simulink model "pend2"  (R2017b)
settings: Solver=VariableStepAuto  StartTime=0.0  StopTime=1  RelTol=1e-3
libraries: simulink_extras x6, simulink x2
settings Model: Creator=Iman  LastModifiedBy=Iman

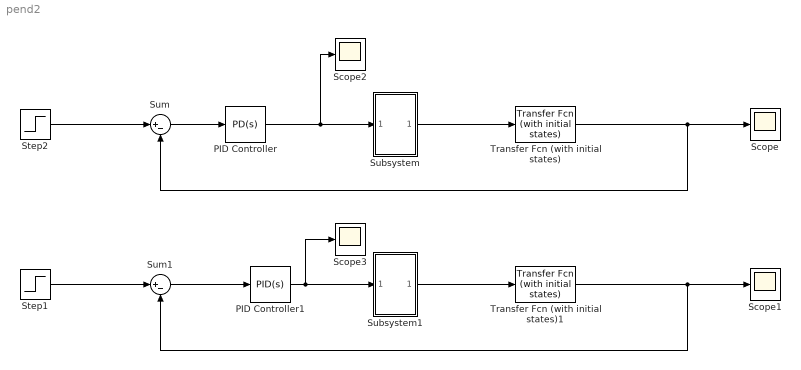
== system pend2 ==
  PID Controller : simulink/Continuous/PID Controller  Controller=PD  TimeDomain=Continuous-time  SampleTime=-1  IntegratorMethod=Forward Euler  FilterMethod=Forward Euler  Form=Parallel  UseFilter=on  ControllerParametersSource=internal  P=-1149.38229083247  I=-498.232243634702  D=-2.84895426178674  N=145.911718528072  InitialConditionSource=internal  InitialConditionForIntegrator=0  InitialConditionForFilter=0  ExternalReset=none  LimitOutput=off  UpperSaturationLimit=inf  LowerSaturationLimit=-inf  LinearizeAsGain=on  AntiWindupMode=none  Kb=1  TrackingMode=off  Kt=1  PParamMin=[]  PParamMax=[]  IParamMin=[]  IParamMax=[]  DParamMin=[]  DParamMax=[]  NParamMin=[]  NParamMax=[]  KbParamMin=[]  KbParamMax=[]  KtParamMin=[]  KtParamMax=[]  POutMin=[]  POutMax=[]  IOutMin=[]  IOutMax=[]  DOutMin=[]  DOutMax=[]  NOutMin=[]  NOutMax=[]  KbOutMin=[]  KbOutMax=[]  KtOutMin=[]  KtOutMax=[]  IntegratorOutMin=[]  IntegratorOutMax=[]  FilterOutMin=[]  FilterOutMax=[]  SumOutMin=[]  SumOutMax=[]  SumI1OutMin=[]  SumI1OutMax=[]  SumI2OutMin=[]  SumI2OutMax=[]  SumI3OutMin=[]  SumI3OutMax=[]  SumDOutMin=[]  SumDOutMax=[]  SaturationOutMin=[]  SaturationOutMax=[]  IntegratorContinuousStateAttributes=''  IntegratorStateMustResolveToSignalObject=off  IntegratorRTWStateStorageClass=Auto  FilterContinuousStateAttributes=''  FilterStateMustResolveToSignalObject=off  FilterRTWStateStorageClass=Auto  DifferentiatorICPrevScaledInput=0  DifferentiatorOutMin=[]  DifferentiatorOutMax=[]  InitialConditionSetting=State (most efficient)  FilterDiffOutCoefMin=[]  FilterDiffOutCoefMax=[]  SumDenOutMin=[]  SumDenOutMax=[]  SumNumOutMin=[]  SumNumOutMax=[]  ReciprocalOutMin=[]  ReciprocalOutMax=[]  DivideOutMin=[]  DivideOutMax=[]  TunerSelectOption=Transfer Function Based (PID Tuner App)
  PID Controller1 : simulink/Continuous/PID Controller  Controller=PID  TimeDomain=Continuous-time  SampleTime=-1  IntegratorMethod=Forward Euler  FilterMethod=Forward Euler  Form=Parallel  UseFilter=on  ControllerParametersSource=internal  P=50303643.3579245  I=36418344513.5141  D=15438.3063033628  N=14182098.2865599  InitialConditionSource=internal  InitialConditionForIntegrator=0  InitialConditionForFilter=0  ExternalReset=none  LimitOutput=off  UpperSaturationLimit=inf  LowerSaturationLimit=-inf  LinearizeAsGain=on  AntiWindupMode=none  Kb=1  TrackingMode=off  Kt=1  PParamMin=[]  PParamMax=[]  IParamMin=[]  IParamMax=[]  DParamMin=[]  DParamMax=[]  NParamMin=[]  NParamMax=[]  KbParamMin=[]  KbParamMax=[]  KtParamMin=[]  KtParamMax=[]  POutMin=[]  POutMax=[]  IOutMin=[]  IOutMax=[]  DOutMin=[]  DOutMax=[]  NOutMin=[]  NOutMax=[]  KbOutMin=[]  KbOutMax=[]  KtOutMin=[]  KtOutMax=[]  IntegratorOutMin=[]  IntegratorOutMax=[]  FilterOutMin=[]  FilterOutMax=[]  SumOutMin=[]  SumOutMax=[]  SumI1OutMin=[]  SumI1OutMax=[]  SumI2OutMin=[]  SumI2OutMax=[]  SumI3OutMin=[]  SumI3OutMax=[]  SumDOutMin=[]  SumDOutMax=[]  SaturationOutMin=[]  SaturationOutMax=[]  IntegratorContinuousStateAttributes=''  IntegratorStateMustResolveToSignalObject=off  IntegratorRTWStateStorageClass=Auto  FilterContinuousStateAttributes=''  FilterStateMustResolveToSignalObject=off  FilterRTWStateStorageClass=Auto  DifferentiatorICPrevScaledInput=0  DifferentiatorOutMin=[]  DifferentiatorOutMax=[]  InitialConditionSetting=State (most efficient)  FilterDiffOutCoefMin=[]  FilterDiffOutCoefMax=[]  SumDenOutMin=[]  SumDenOutMax=[]  SumNumOutMin=[]  SumNumOutMax=[]  ReciprocalOutMin=[]  ReciprocalOutMax=[]  DivideOutMin=[]  DivideOutMax=[]  TunerSelectOption=Transfer Function Based (PID Tuner App)
  Scope{,1..3} (4 alike) : Scope
  Step1 : Step  Time=0  SampleTime=0.1
  Step2 : Step  Time=0  After=0.01  SampleTime=0.1
  Subsystem : Subsystem
  Subsystem1 : Subsystem
  Sum : Sum  Inputs=|+-
  Sum1 : Sum  Inputs=|+-
  Transfer Fcn (with initial states) : simulink_extras/Additional Linear/Transfer Fcn (with initial states)  N=[-1374 -7.66e04]  D=[1 2549 -370.1 -1.28e05]  X0=0
  Transfer Fcn (with initial states)1 : simulink_extras/Additional Linear/Transfer Fcn (with initial states)  N=[104.5 -3064 -6898]  D=[1 2549 -370.1 -1.28e05 0]  X0=0
  wires:
  Transfer Fcn (with initial states)/1 -> Sum/2, Scope/1
  Step2/1 -> Sum/1
  Sum/1 -> PID Controller/1
  PID Controller/1 -> Scope2/1, Subsystem/1(In1)
  Subsystem/1(Out1) -> Transfer Fcn (with initial states)/1
  Transfer Fcn (with initial states)1/1 -> Sum1/2, Scope1/1
  PID Controller1/1 -> Scope3/1, Subsystem1/1(In1)
  Subsystem1/1(Out1) -> Transfer Fcn (with initial states)1/1
  Step1/1 -> Sum1/1
  Sum1/1 -> PID Controller1/1

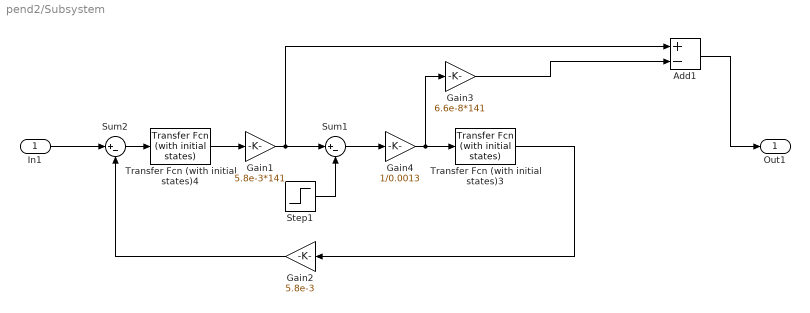
== system pend2/Subsystem ==
  In1 : Inport
  Add1 : Sum  Inputs=+-
  Gain1 : Gain  Gain=5.8e-3*141
  Gain2 : Gain  Gain=5.8e-3
  Gain3 : Gain  Gain=6.6e-8*141
  Gain4 : Gain  Gain=1/0.0013
  Step1 : Step  Time=0  SampleTime=0.1
  Sum1 : Sum  Inputs=|+-
  Sum2 : Sum  Inputs=|+-
  Transfer Fcn (with initial states)3 : simulink_extras/Additional Linear/Transfer Fcn (with initial states)  N=[1]  D=[1 0]  X0=0
  Transfer Fcn (with initial states)4 : simulink_extras/Additional Linear/Transfer Fcn (with initial states)  N=[1]  D=[7e-5 6]  X0=0
  Out1 : Outport
  wires:
  Transfer Fcn (with initial states)3/1 -> Gain2/1
  Step1/1 -> Sum1/2
  Sum1/1 -> Gain4/1
  Add1/1 -> Out1/1
  Gain1/1 -> Sum1/1, Add1/1
  Gain2/1 -> Sum2/2
  Transfer Fcn (with initial states)4/1 -> Gain1/1
  Gain3/1 -> Add1/2
  Gain4/1 -> Gain3/1, Transfer Fcn (with initial states)3/1
  Sum2/1 -> Transfer Fcn (with initial states)4/1
  In1/1 -> Sum2/1

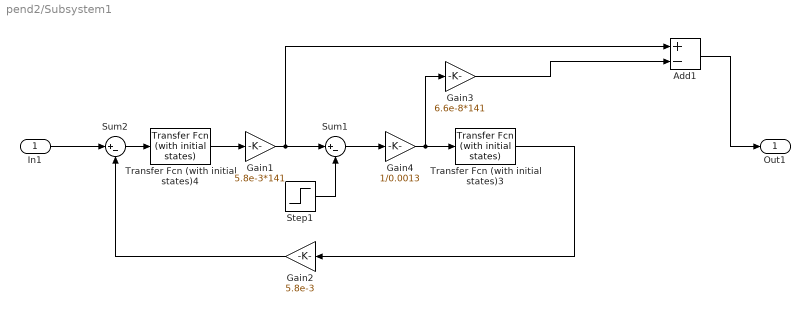
== system pend2/Subsystem1 ==
  In1 : Inport
  Add1 : Sum  Inputs=+-
  Gain1 : Gain  Gain=5.8e-3*141
  Gain2 : Gain  Gain=5.8e-3
  Gain3 : Gain  Gain=6.6e-8*141
  Gain4 : Gain  Gain=1/0.0013
  Step1 : Step  Time=0  SampleTime=0.1
  Sum1 : Sum  Inputs=|+-
  Sum2 : Sum  Inputs=|+-
  Transfer Fcn (with initial states)3 : simulink_extras/Additional Linear/Transfer Fcn (with initial states)  N=[1]  D=[1 0]  X0=0
  Transfer Fcn (with initial states)4 : simulink_extras/Additional Linear/Transfer Fcn (with initial states)  N=[1]  D=[7e-5 6]  X0=0
  Out1 : Outport
  wires:
  Transfer Fcn (with initial states)3/1 -> Gain2/1
  Step1/1 -> Sum1/2
  Sum1/1 -> Gain4/1
  Add1/1 -> Out1/1
  Gain1/1 -> Sum1/1, Add1/1
  Gain2/1 -> Sum2/2
  Transfer Fcn (with initial states)4/1 -> Gain1/1
  Gain3/1 -> Add1/2
  Gain4/1 -> Gain3/1, Transfer Fcn (with initial states)3/1
  Sum2/1 -> Transfer Fcn (with initial states)4/1
  In1/1 -> Sum2/1
